simulink model "TASK8_2"  (R2019a)
settings: Solver=VariableStepAuto  StartTime=0.0  StopTime=30  RelTol=1e-3
values from neighbouring files (symbols this model uses):
  A = [0,mf*g*h/Jconst,0,-(mf*g)/Jconst;1,0,0,0;0,-g,0,0;0,0,1,0]    [Dharmesh_DCS_LAB_Script.m]
  B = [1/Jconst;0;0;0]    [Dharmesh_DCS_LAB_Script.m]
  C = eye(4)    [Dharmesh_DCS_LAB_Script.m]
  Ct = [0 0 0 1]    [Dharmesh_DCS_LAB_Script.m]
  D = [0;0;0;0]    [Dharmesh_DCS_LAB_Script.m]
  Kpi = qI*(alpha(6)*eye(5) + alpha(5)*Api + alpha(4)*Api^2 + alpha(3)*Api^3 + alpha(2)*Api^4 + alpha(1)*Api^5)    [Dharmesh_DCS_LAB_Script.m]
  Kt_o_new = Kt_o.'    [Dharmesh_DCS_LAB_Script.m]
  P = 1/(Ct*inv((B*K)-A)*B)    [Dharmesh_DCS_LAB_Script.m]
  Pi = -Kpi(5)    [Dharmesh_DCS_LAB_Script.m]
  Ts = 125e-6    (= 0.000125)    [Dharmesh_DCS_LAB_Script.m]
undefined symbols (not defined in the file or in its folder): AD, BD
settings Model: Creator=Admin  LastModifiedBy=Admin

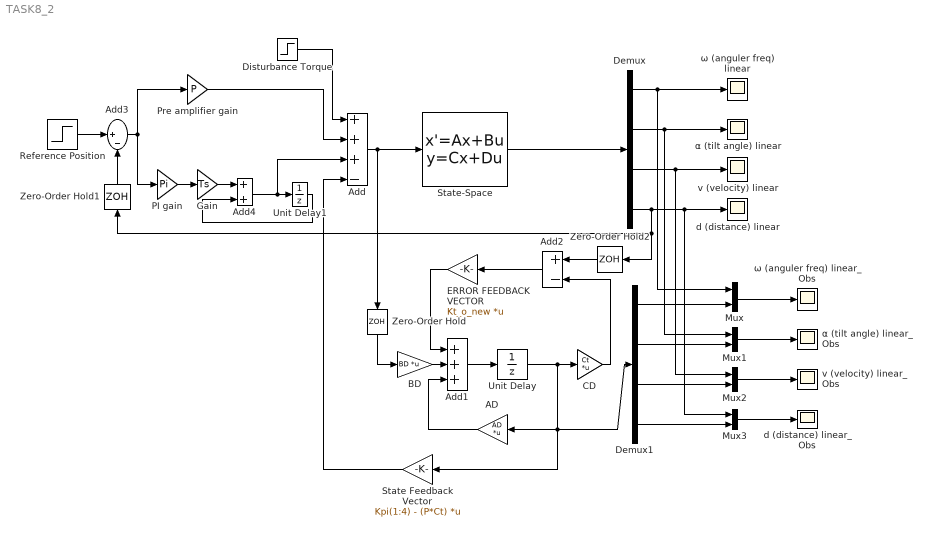
== system TASK8_2 ==
  AD : Gain  Gain=AD  Multiplication=Matrix(K*u) (u vector)
  Add : Sum  Inputs=+++-
  Add1 : Sum  Inputs=+++
  Add2 : Sum  Inputs=+-
  Add3 : Sum  Inputs=|+-
  Add4 : Sum
  BD : Gain  Gain=BD  Multiplication=Matrix(K*u) (u vector)
  CD : Gain  Gain=Ct  Multiplication=Matrix(K*u) (u vector)
  Demux : Demux
  Demux1 : Demux
  Disturbance Torque : Step  Time=15  After=0.1  SampleTime=0
  ERROR FEEDBACK VECTOR : Gain  Gain=Kt_o_new  Multiplication=Matrix(K*u) (u vector)
  Gain : Gain  Gain=Ts
  Mux{,1..3} (4 alike) : Mux  Inputs=2
  PI gain : Gain  Gain=Pi
  Pre amplifier gain : Gain  Gain=P
  Reference Position : Step  Time=0  SampleTime=0
  State Feedback Vector : Gain  Gain=Kpi(1:4) - (P*Ct)  Multiplication=Matrix(K*u) (u vector)
  State-Space : StateSpace  A=A  B=B  C=C  D=D  InitialCondition=0
  Unit Delay : UnitDelay  InitialCondition=[0;0;0;1]  SampleTime=Ts  HasFrameUpgradeWarning=on
  Unit Delay1 : UnitDelay  SampleTime=Ts  HasFrameUpgradeWarning=on
  Zero-Order Hold : ZeroOrderHold  SampleTime=Ts
  Zero-Order Hold1 : ZeroOrderHold  SampleTime=Ts
  Zero-Order Hold2 : ZeroOrderHold  SampleTime=Ts
  d (distance) linear : Scope
  d (distance) linear_Obs : Scope
  v (velocity) linear : Scope
  v (velocity) linear_Obs : Scope
  α (tilt angle) linear : Scope
  α (tilt angle) linear_Obs : Scope
  ω (anguler freq) linear : Scope
  ω (anguler freq) linear_Obs : Scope
  wires:
  Mux2/1 -> v (velocity) linear_Obs/1
  Demux1/3 -> Mux2/2
  Demux1/1 -> Mux/2
  Demux1/2 -> Mux1/2
  Mux/1 -> ω (anguler freq) linear_Obs/1
  Mux1/1 -> α (tilt angle) linear_Obs/1
  State Feedback Vector/1 -> Add/4
  AD/1 -> Add1/3
  BD/1 -> Add1/2
  Demux1/4 -> Mux3/2
  Add/1 -> State-Space/1, Zero-Order Hold/1
  State-Space/1 -> Demux/1
  Demux/1 -> Mux/1, ω (anguler freq) linear/1
  ERROR FEEDBACK VECTOR/1 -> Add1/1
  Demux/3 -> Mux2/1, v (velocity) linear/1
  Demux/2 -> Mux1/1, α (tilt angle) linear/1
  Add2/1 -> ERROR FEEDBACK VECTOR/1
  Pre amplifier gain/1 -> Add/2
  Unit Delay/1 -> Demux1/1, AD/1, State Feedback Vector/1, CD/1
  Add1/1 -> Unit Delay/1
  Mux3/1 -> d (distance) linear_Obs/1
  Demux/4 -> Zero-Order Hold1/1, Zero-Order Hold2/1, Mux3/1, d (distance) linear/1
  CD/1 -> Add2/2
  Zero-Order Hold/1 -> BD/1
  Reference Position/1 -> Add3/1
  Zero-Order Hold1/1 -> Add3/2
  Zero-Order Hold2/1 -> Add2/1
  Disturbance Torque/1 -> Add/1
  Add3/1 -> PI gain/1, Pre amplifier gain/1
  Add4/1 -> Add/3, Unit Delay1/1
  Unit Delay1/1 -> Add4/2
  PI gain/1 -> Gain/1
  Gain/1 -> Add4/1
